simulink model "nms_model"  (R2020a)
settings: Solver=ode15s  StartTime=0.0  StopTime=2.6  MaxStep=.01  RelTol=1e-4  AbsTol=1e-6  EnableMultiTasking=on
values from neighbouring files (symbols this model uses):
  dt_visual = -1    [NMScontrol.m]    (also in runmodel.m = 0.001)
  g = params.g    [NMPCcostFunction.m]    (also in dynamicsNMPC.m = 9.81)
  m = parametersOpt(1)    [CGBgreybox.m]    (also in NMPCcostFunction.m = params.m)
undefined symbols (not defined in the file or in its folder): hatLeftHipToCenterDistWidth, initialTargetAngle, LongDelay, LongLoopDelay, LPreStimBFSHinit, LPreStimGASinit, LPreStimGLUinit, LPreStimHABinit, LPreStimHADinit, LPreStimHAMinit, LPreStimHFLinit, LPreStimRFinit, LPreStimSOLinit, LPreStimTAinit, LPreStimVASinit, LTargetAngleInit, LTargetAngleRInit, MidDelay, RPreStimBFSHinit, RPreStimGASinit, RPreStimGLUinit, RPreStimHABinit, RPreStimHADinit, RPreStimHAMinit, RPreStimHFLinit, RPreStimRFinit, RPreStimSOLinit, RPreStimTAinit, RPreStimVASinit, RTargetAngleInit, RTargetAngleRInit, ShortDelay, termination_height, thetaHATref, X, Y, Z
libraries: NeuroMuscularLibrary x107, nesl_utility x25, sm_lib x16, simulink x3
(part 2 of 3)

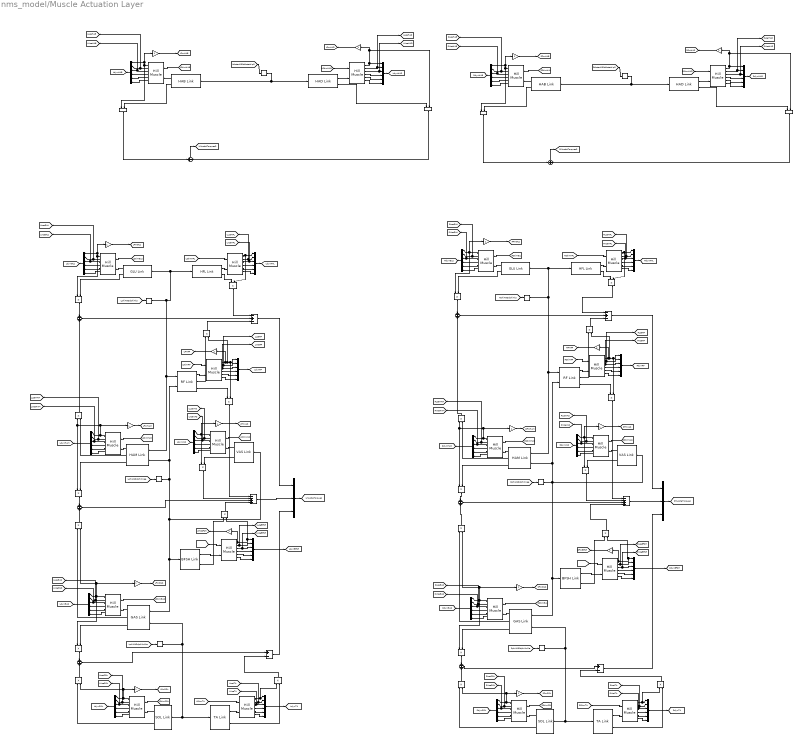
== system nms_model/Muscle Actuation Layer ==
  note: Right Hip Joint
  note: Right Knee Joint
  note: Right Ankle Joint
  note: Left Hip Joint
  note: Left Knee Joint
  note: Left Ankle Joint
  note: Left Leg
  note: Right Leg
  note: Body Mechanics Layer
      | Interface (Left Hip Joint)
  note: Muscle Actuation Layer
      | (Coronal Plane)
  note: Muscle Actuation Layer
      | (Sagittal Plane)
  note: Body Mechanics Layer
      | Interface (Right Hip Joint)
  Add1 : Sum  Inputs=-+-
  Add2 : Sum  Inputs=-+-
  Add3 : Sum  Inputs=--++
  Add4 : Sum  Inputs=+-
  Add5 : Sum  Inputs=--++
  Add6 : Sum  Inputs=+-
  L  TA Link : NeuroMuscularLibrary/TA Link  SystemSampleTime=-1  Latency=0  AutoFrameSizeCalculation=off
  L BFSH Golgi Tendon Organs : Gain
  L BFSH Link : NeuroMuscularLibrary/BFSH Link  SystemSampleTime=-1  Latency=0  AutoFrameSizeCalculation=off
  L BFSH Muscle : NeuroMuscularLibrary/Hill Muscle  Fmax=FmaxBFSH  lopt=loptBFSH  vmax=vmaxBFSH  lslack=lslackBFSH
  L GAS Golgi Tendon Organs : Gain
  L GAS Link : NeuroMuscularLibrary/GAS Link  SystemSampleTime=-1  Latency=0  AutoFrameSizeCalculation=off
  L GAS Muscle : NeuroMuscularLibrary/Hill Muscle  Fmax=FmaxGAS  lopt=loptGAS  vmax=vmaxGAS  lslack=lslackGAS
  L GLU Golgi Tendon Organs : Gain
  L GLU Link : NeuroMuscularLibrary/GLU Link  SystemSampleTime=-1  Latency=0  AutoFrameSizeCalculation=off
  L GLU Muscle : NeuroMuscularLibrary/Hill Muscle  Fmax=FmaxGLU  lopt=loptGLU  vmax=vmaxGLU  lslack=lslackGLU
  L HAB Golgi Tendon Organs : Gain
  L HAB Link : NeuroMuscularLibrary/HAB Link  SystemSampleTime=-1  Latency=0  AutoFrameSizeCalculation=off
  L HAB Muscle : NeuroMuscularLibrary/Hill Muscle  Fmax=FmaxHAB  lopt=loptHAB  vmax=vmaxHAB  lslack=lslackHAB
  L HAD Golgi Tendon Organs : Gain
  L HAD Link : NeuroMuscularLibrary/HAD Link  SystemSampleTime=-1  Latency=0  AutoFrameSizeCalculation=off
  L HAD Muscle : NeuroMuscularLibrary/Hill Muscle  Fmax=FmaxHAD  lopt=loptHAD  vmax=vmaxHAD  lslack=lslackHAD
  L HAM Golgi Tendon Organs : Gain
  L HAM Link : NeuroMuscularLibrary/HAM Link  SystemSampleTime=-1  Latency=0  AutoFrameSizeCalculation=off
  L HAM Muscle : NeuroMuscularLibrary/Hill Muscle  Fmax=FmaxHAM  lopt=loptHAM  vmax=vmaxHAM  lslack=lslackHAM
  L HFL Link : NeuroMuscularLibrary/HFL Link  SystemSampleTime=-1  Latency=0  AutoFrameSizeCalculation=off
  L HFL Muscle : NeuroMuscularLibrary/Hill Muscle  Fmax=FmaxHFL  lopt=loptHFL  vmax=vmaxHFL  lslack=lslackHFL
  L RF Golgi Tendon Organs : Gain
  L RF Link : NeuroMuscularLibrary/RF Link  SystemSampleTime=-1  Latency=0  AutoFrameSizeCalculation=off
  L RF Muscle : NeuroMuscularLibrary/Hill Muscle  Fmax=FmaxRF  lopt=loptRF  vmax=vmaxRF  lslack=lslackRF
  L SOL Golgi Tendon Organs : Gain
  L SOL Link : NeuroMuscularLibrary/SOL Link  SystemSampleTime=-1  Latency=0  AutoFrameSizeCalculation=off
  L SOL Muscle : NeuroMuscularLibrary/Hill Muscle  Fmax=FmaxSOL  lopt=loptSOL  vmax=vmaxSOL  lslack=lslackSOL
  L TA Muscle : NeuroMuscularLibrary/Hill Muscle  Fmax=FmaxTA  lopt=loptTA  vmax=vmaxTA  lslack=lslackTA
  L VAS Golgi Tendon Organs : Gain
  L VAS Link : NeuroMuscularLibrary/VAS Link  SystemSampleTime=-1  Latency=0  AutoFrameSizeCalculation=off
  L VAS Muscle : NeuroMuscularLibrary/Hill Muscle  Fmax=FmaxVAS  lopt=loptVAS  vmax=vmaxVAS  lslack=lslackVAS
  Mux : Mux  Inputs=3
  Mux1 : Mux  Inputs=3
  Mux{2..23} (22 alike) : Mux  Inputs=6
  Product{1..2,26..27} (4 alike) : Product  RndMeth=Zero
  R  TA Link : NeuroMuscularLibrary/TA Link  SystemSampleTime=-1  Latency=0  AutoFrameSizeCalculation=off
  R BFSH Golgi Tendon Organs : Gain
  R BFSH Link : NeuroMuscularLibrary/BFSH Link  SystemSampleTime=-1  Latency=0  AutoFrameSizeCalculation=off
  R BFSH Muscle : NeuroMuscularLibrary/Hill Muscle  Fmax=FmaxBFSH  lopt=loptBFSH  vmax=vmaxBFSH  lslack=lslackBFSH
  R GAS Golgi Tendon Organs : Gain
  R GAS Link : NeuroMuscularLibrary/GAS Link  SystemSampleTime=-1  Latency=0  AutoFrameSizeCalculation=off
  R GAS Muscle : NeuroMuscularLibrary/Hill Muscle  Fmax=FmaxGAS  lopt=loptGAS  vmax=vmaxGAS  lslack=lslackGAS
  R GLU Golgi Tendon Organs : Gain
  R GLU Link : NeuroMuscularLibrary/GLU Link  SystemSampleTime=-1  Latency=0  AutoFrameSizeCalculation=off
  R GLU Muscle : NeuroMuscularLibrary/Hill Muscle  Fmax=FmaxGLU  lopt=loptGLU  vmax=vmaxGLU  lslack=lslackGLU
  R HAB Golgi Tendon Organs : Gain
  R HAB Link : NeuroMuscularLibrary/HAB Link  SystemSampleTime=-1  Latency=0  AutoFrameSizeCalculation=off
  R HAB Muscle : NeuroMuscularLibrary/Hill Muscle  Fmax=FmaxHAB  lopt=loptHAB  vmax=vmaxHAB  lslack=lslackHAB
  R HAD Golgi Tendon Organs : Gain
  R HAD Link : NeuroMuscularLibrary/HAD Link  SystemSampleTime=-1  Latency=0  AutoFrameSizeCalculation=off
  R HAD Muscle : NeuroMuscularLibrary/Hill Muscle  Fmax=FmaxHAD  lopt=loptHAD  vmax=vmaxHAD  lslack=lslackHAD
  R HAM Golgi Tendon Organs : Gain
  R HAM Link : NeuroMuscularLibrary/HAM Link  SystemSampleTime=-1  Latency=0  AutoFrameSizeCalculation=off
  R HAM Muscle : NeuroMuscularLibrary/Hill Muscle  Fmax=FmaxHAM  lopt=loptHAM  vmax=vmaxHAM  lslack=lslackHAM
  R HFL Link : NeuroMuscularLibrary/HFL Link  SystemSampleTime=-1  Latency=0  AutoFrameSizeCalculation=off
  R HFL Muscle : NeuroMuscularLibrary/Hill Muscle  Fmax=FmaxHFL  lopt=loptHFL  vmax=vmaxHFL  lslack=lslackHFL
  R RF Golgi Tendon Organs : Gain
  R RF Link : NeuroMuscularLibrary/RF Link  SystemSampleTime=-1  Latency=0  AutoFrameSizeCalculation=off
  R RF Muscle : NeuroMuscularLibrary/Hill Muscle  Fmax=FmaxRF  lopt=loptRF  vmax=vmaxRF  lslack=lslackRF
  R SOL Golgi Tendon Organs : Gain
  R SOL Link : NeuroMuscularLibrary/SOL Link  SystemSampleTime=-1  Latency=0  AutoFrameSizeCalculation=off
  R SOL Muscle : NeuroMuscularLibrary/Hill Muscle  Fmax=FmaxSOL  lopt=loptSOL  vmax=vmaxSOL  lslack=lslackSOL
  R TA Muscle : NeuroMuscularLibrary/Hill Muscle  Fmax=FmaxTA  lopt=loptTA  vmax=vmaxTA  lslack=lslackTA
  R VAS Golgi Tendon Organs : Gain
  R VAS Link : NeuroMuscularLibrary/VAS Link  SystemSampleTime=-1  Latency=0  AutoFrameSizeCalculation=off
  R VAS Muscle : NeuroMuscularLibrary/Hill Muscle  Fmax=FmaxVAS  lopt=loptVAS  vmax=vmaxVAS  lslack=lslackVAS
  Selector{1..8} (8 alike) : Selector  InputPortWidth=2  IndexOptions=Index vector (dialog)  Indices=1  OutputSizes=1
  Sum{1,3..4,8,11,15} (6 alike) : Sum  Inputs=+|+
  Sum2 : Sum  Inputs=+-
  Sum25 : Sum  Inputs=+-
  tau = r*F{1..24} (24 alike) : Product
  tag scope: LFmBFSH=global, LFmGAS=global, LFmGLU=global, LFmHAB=global, LFmHAD=global, LFmHAM=global, LFmRF=global, LFmSOL=global, LFmVAS=global, LLceBFSH=global, LLceGAS=global, LLceGLU=global, LLceHAB=global, LLceHAD=global, LLceHAM=global, LLceHFL=global, LLceRF=global, LLceSOL=global, LLceTA=global, LLceVAS=global, LMuscleTorques=global, LMuscleTorquesR=global, LVceBFSH=global, LVceGAS=global, LVceGLU=global, LVceHAB=global, LVceHAD=global, LVceHAM=global, LVceHFL=global, LVceRF=global, LVceSOL=global, LVceTA=global, LVceVAS=global, LdynBFSH=global, LdynGAS=global, LdynGLU=global, LdynHAB=global, LdynHAD=global, LdynHAM=global, LdynHFL=global, LdynRF=global, LdynSOL=global, LdynTA=global, LdynVAS=global, RFmBFSH=global, RFmGAS=global, RFmGLU=global, RFmHAB=global, RFmHAD=global, RFmHAM=global, RFmRF=global, RFmSOL=global, RFmVAS=global, RLceBFSH=global, RLceGAS=global, RLceGLU=global, RLceHAB=global, RLceHAD=global, RLceHAM=global, RLceHFL=global, RLceRF=global, RLceSOL=global, RLceTA=global, RLceVAS=global, RMuscleTorques=global, RMuscleTorquesR=global, RVceBFSH=global, RVceGAS=global, RVceGLU=global, RVceHAB=global, RVceHAD=global, RVceHAM=global, RVceHFL=global, RVceRF=global, RVceSOL=global, RVceTA=global, RVceVAS=global, RdynBFSH=global, RdynGAS=global, RdynGLU=global, RdynHAB=global, RdynHAD=global, RdynHAM=global, RdynHFL=global, RdynRF=global, RdynSOL=global, RdynTA=global, RdynVAS=global
  wires:
  R HAM Link/1 -> R HAM Muscle/2
  R HAM Link/2 -> tau = r*F9/2
  R HAM Muscle/5 -> Mux7/5
  Mux7/1 -> [RdynHAM]
  R HAM Muscle/3 -> [RVceHAM], Mux7/3
  R HAM Muscle/4 -> Mux7/4
  [RphiANDdphiHip] -> Selector1/1
  Selector1/1 -> R RF Link/1, R HAM Link/1, R GLU Link/1, R HFL Link/1
  Add2/1 -> Mux/1
  R GLU Link/1 -> R GLU Muscle/2
  [RStimGLU] -> R GLU Muscle/1
  R GLU Muscle/5 -> Mux9/5
  R GLU Muscle/2 -> [RLceGLU], Mux9/2
  R GLU Muscle/3 -> [RVceGLU], Mux9/3
  R GLU Muscle/4 -> Mux9/4
  R GLU Link/2 -> tau = r*F10/2
  R GLU Muscle/1 -> Mux9/1, R GLU Golgi Tendon Organs/1, tau = r*F10/1
  R GLU Golgi Tendon Organs/1 -> [RFmGLU]
  R HFL Link/1 -> R HFL Muscle/2
  [RStimHFL] -> R HFL Muscle/1
  R HFL Muscle/5 -> Mux10/5
  Mux10/1 -> [RdynHFL]
  R HFL Muscle/4 -> Mux10/4
  R HFL Muscle/3 -> [RVceHFL], Mux10/3
  R HFL Link/2 -> tau = r*F11/1
  R HFL Muscle/1 -> Mux10/1, tau = r*F11/2
  R HAM Golgi Tendon Organs/1 -> [RFmHAM]
  [RStimHAM] -> R HAM Muscle/1
  R VAS Link/1 -> R VAS Muscle/2
  R VAS Muscle/5 -> Mux11/5
  Mux11/1 -> [RdynVAS]
  R VAS Muscle/2 -> [RLceVAS], Mux11/2
  R VAS Muscle/3 -> [RVceVAS], Mux11/3
  R VAS Muscle/4 -> Mux11/4
  R VAS Muscle/1 -> R VAS Golgi Tendon Organs/1, Mux11/1, tau = r*F13/1
  R VAS Golgi Tendon Organs/1 -> [RFmVAS]
  R VAS Link/2 -> tau = r*F13/2
  R HAM Link/3 -> tau = r*F14/2
  Sum11/1 -> Add3/3  "Knee Flexion Torque"
  [RStimVAS] -> R VAS Muscle/1
  [RphiANDdphiKnee] -> Selector3/1
  R SOL Muscle/1 -> R SOL Golgi Tendon Organs/1, tau = r*F12/2, Mux13/1
  R SOL Muscle/5 -> Mux13/5
  Mux13/1 -> [RdynSOL]
  R SOL Muscle/2 -> [RLceSOL], Mux13/2
  R SOL Muscle/3 -> [RVceSOL], Mux13/3
  R SOL Muscle/4 -> Mux13/4
  R SOL Link/2 -> tau = r*F12/1
  R SOL Link/1 -> R SOL Muscle/2
  R SOL Golgi Tendon Organs/1 -> [RFmSOL]
  [RStimSOL] -> R SOL Muscle/1
  Selector2/1 -> R GAS Link/2, R  TA Link/1, R SOL Link/1
  [RphiANDdphiAnkle] -> Selector2/1
  Add4/1 -> Mux/3
  R  TA Link/1 -> R TA Muscle/2
  R TA Muscle/1 -> tau = r*F15/1, Mux14/1
  R TA Muscle/5 -> Mux14/5
  Mux14/1 -> [RdynTA]
  R TA Muscle/4 -> Mux14/4
  R TA Muscle/3 -> Mux14/3, [RVceTA]
  [RStimTA] -> R TA Muscle/1
  R  TA Link/2 -> tau = r*F15/2
  tau = r*F15/1 -> Add4/2
  R GAS Link/1 -> R GAS Muscle/2
  Selector3/1 -> R RF Link/2, R HAM Link/2, R VAS Link/1, R GAS Link/1, R BFSH Link/1
  R GAS Muscle/5 -> Mux12/5
  Mux12/1 -> [RdynGAS]
  R GAS Muscle/2 -> [RLceGAS], Mux12/2
  R GAS Muscle/3 -> [RVceGAS], Mux12/3
  R GAS Muscle/4 -> Mux12/4
  R GAS Link/2 -> tau = r*F16/1
  [RStimGAS] -> R GAS Muscle/1
  tau = r*F12/1 -> Sum15/2
  Sum15/1 -> Add4/1
  R GAS Link/3 -> tau = r*F17/2
  tau = r*F17/1 -> Sum15/1
  R GAS Muscle/1 -> Mux12/1, tau = r*F16/2, R GAS Golgi Tendon Organs/1, tau = r*F17/1
  R GAS Golgi Tendon Organs/1 -> [RFmGAS]
  tau = r*F9/1 -> Sum8/2  "HAM"
  tau = r*F10/1 -> Sum8/1  "GLU"
  tau = r*F11/1 -> Add2/1  "HFL"
  R HAM Muscle/1 -> tau = r*F14/1, tau = r*F9/1, R HAM Golgi Tendon Organs/1, Mux7/1
  Sum8/1 -> Add2/2  "Hip Extension Moment"
  tau = r*F16/1 -> Sum11/2  "GAS"
  tau = r*F14/1 -> Sum11/1  "HAM"
  tau = r*F13/1 -> Add3/2  "VAS"
  R TA Muscle/2 -> [RLceTA], Mux14/2
  Mux9/1 -> [RdynGLU]
  Mux/1 -> [RMuscleTorques]
  L HAM Link/1 -> L HAM Muscle/2
  L HAM Link/2 -> tau = r*F18/2
  L HAM Muscle/5 -> Mux8/5
  Mux8/1 -> [LdynHAM]
  L HAM Muscle/3 -> [LVceHAM], Mux8/3
  L HAM Muscle/4 -> Mux8/4
  [LphiANDdphiHip] -> Selector4/1
  Selector4/1 -> L GLU Link/1, L HFL Link/1, L RF Link/1, L HAM Link/1
  Add1/1 -> Mux1/1
  L GLU Link/1 -> L GLU Muscle/2
  [LStimGLU] -> L GLU Muscle/1
  L GLU Muscle/5 -> Mux15/5
  L GLU Muscle/2 -> Mux15/2, [LLceGLU]
  L GLU Muscle/3 -> Mux15/3, [LVceGLU]
  L GLU Muscle/4 -> Mux15/4
  L GLU Link/2 -> tau = r*F1/2
  L GLU Muscle/1 -> Mux15/1, L GLU Golgi Tendon Organs/1, tau = r*F1/1
  L GLU Golgi Tendon Organs/1 -> [LFmGLU]
  L HFL Link/1 -> L HFL Muscle/2
  [LStimHFL] -> L HFL Muscle/1
  L HFL Muscle/5 -> Mux2/5
  Mux2/1 -> [LdynHFL]
  L HFL Muscle/4 -> Mux2/4
  L HFL Muscle/3 -> [LVceHFL], Mux2/3
  L HFL Link/2 -> tau = r*F2/1
  L HFL Muscle/1 -> Mux2/1, tau = r*F2/2
  L HAM Golgi Tendon Organs/1 -> [LFmHAM]
  [LStimHAM] -> L HAM Muscle/1
  L VAS Link/1 -> L VAS Muscle/2
  L VAS Muscle/5 -> Mux3/5
  Mux3/1 -> [LdynVAS]
  L VAS Muscle/2 -> [LLceVAS], Mux3/2
  L VAS Muscle/3 -> [LVceVAS], Mux3/3
  L VAS Muscle/4 -> Mux3/4
  L VAS Muscle/1 -> L VAS Golgi Tendon Organs/1, Mux3/1, tau = r*F4/1
  L VAS Golgi Tendon Organs/1 -> [LFmVAS]
  L VAS Link/2 -> tau = r*F4/2
  L HAM Link/3 -> tau = r*F5/2
  Sum1/1 -> Add5/3  "Knee Flexion Torque"
  [LStimVAS] -> L VAS Muscle/1
  [LphiANDdphiKnee] -> Selector6/1
  L SOL Muscle/1 -> L SOL Golgi Tendon Organs/1, tau = r*F3/2, Mux5/1
  L SOL Muscle/5 -> Mux5/5
  Mux5/1 -> [LdynSOL]
  L SOL Muscle/3 -> [LVceSOL], Mux5/3
  L SOL Muscle/4 -> Mux5/4
  L SOL Link/2 -> tau = r*F3/1
  L SOL Link/1 -> L SOL Muscle/2
  L SOL Golgi Tendon Organs/1 -> [LFmSOL]
  [LStimSOL] -> L SOL Muscle/1
  Selector5/1 -> L GAS Link/2, L  TA Link/1, L SOL Link/1
  [LphiANDdphiAnkle] -> Selector5/1
  Add6/1 -> Mux1/3
  L  TA Link/1 -> L TA Muscle/2
  L TA Muscle/1 -> tau = r*F6/1, Mux6/1
  L TA Muscle/5 -> Mux6/5
  Mux6/1 -> [LdynTA]
  L TA Muscle/4 -> Mux6/4
  L TA Muscle/3 -> Mux6/3, [LVceTA]
  [LStimTA] -> L TA Muscle/1
  L  TA Link/2 -> tau = r*F6/2
  tau = r*F6/1 -> Add6/2
  L GAS Link/1 -> L GAS Muscle/2
  Selector6/1 -> L GAS Link/1, L BFSH Link/1, L VAS Link/1, L RF Link/2, L HAM Link/2
  L GAS Muscle/5 -> Mux4/5
  Mux4/1 -> [LdynGAS]
  L GAS Muscle/2 -> [LLceGAS], Mux4/2
  L GAS Muscle/3 -> [LVceGAS], Mux4/3
  L GAS Muscle/4 -> Mux4/4
  L GAS Link/2 -> tau = r*F7/1
  [LStimGAS] -> L GAS Muscle/1
  tau = r*F3/1 -> Sum3/2
  Sum3/1 -> Add6/1
  L GAS Link/3 -> tau = r*F8/2
  tau = r*F8/1 -> Sum3/1
  L GAS Muscle/1 -> Mux4/1, tau = r*F7/2, L GAS Golgi Tendon Organs/1, tau = r*F8/1
  L GAS Golgi Tendon Organs/1 -> [LFmGAS]
  tau = r*F18/1 -> Sum4/2  "HAM"
  tau = r*F1/1 -> Sum4/1  "GLU"
  tau = r*F2/1 -> Add1/1  "HFL"
  L HAM Muscle/1 -> tau = r*F5/1, tau = r*F18/1, L HAM Golgi Tendon Organs/1, Mux8/1
  Sum4/1 -> Add1/2  "Hip Extension Moment"
  tau = r*F7/1 -> Sum1/2  "GAS"
  tau = r*F5/1 -> Sum1/1  "HAM"
  tau = r*F4/1 -> Add5/2  "VAS"
  L TA Muscle/2 -> [LLceTA], Mux6/2
  Mux15/1 -> [LdynGLU]
  Mux1/1 -> [LMuscleTorques]
  L GLU Muscle/6 -> Mux15/6
  L HFL Muscle/6 -> Mux2/6
  L HAM Muscle/6 -> Mux8/6
  L VAS Muscle/6 -> Mux3/6
  L GAS Muscle/6 -> Mux4/6
  L SOL Muscle/6 -> Mux5/6
  L TA Muscle/6 -> Mux6/6
  R SOL Muscle/6 -> Mux13/6
  R TA Muscle/6 -> Mux14/6
  R GAS Muscle/6 -> Mux12/6
  R HAM Muscle/6 -> Mux7/6
  R VAS Muscle/6 -> Mux11/6
  R HFL Muscle/6 -> Mux10/6
  R GLU Muscle/6 -> Mux9/6
  R HFL Muscle/2 -> [RLceHFL], Mux10/2
  R HAM Muscle/2 -> [RLceHAM], Mux7/2
  L HFL Muscle/2 -> [LLceHFL], Mux2/2
  L HAM Muscle/2 -> [LLceHAM], Mux8/2
  L SOL Muscle/2 -> [LLceSOL], Mux5/2
  L BFSH Muscle/3 -> [LVceBFSH], Mux16/3
  [LStimBFSH] -> L BFSH Muscle/1
  L BFSH Link/2 -> tau = r*F19/1
  L BFSH Golgi Tendon Organs/1 -> [LFmBFSH]
  L BFSH Muscle/6 -> Mux16/6
  L BFSH Muscle/4 -> Mux16/4
  L BFSH Link/1 -> L BFSH Muscle/2
  Mux16/1 -> [LdynBFSH]
  L BFSH Muscle/2 -> [LLceBFSH], Mux16/2
  L BFSH Muscle/5 -> Mux16/5
  L BFSH Muscle/1 -> tau = r*F19/2, Mux16/1, L BFSH Golgi Tendon Organs/1
  tau = r*F19/1 -> Add5/4  "BFSH"
  L RF Muscle/3 -> [LVceRF], Mux17/3
  [LStimRF] -> L RF Muscle/1
  L RF Link/3 -> tau = r*F20/2
  L RF Golgi Tendon Organs/1 -> [LFmRF]
  L RF Muscle/6 -> Mux17/6
  L RF Muscle/4 -> Mux17/4
  L RF Link/1 -> L RF Muscle/2
  Mux17/1 -> [LdynRF]
  L RF Muscle/2 -> [LLceRF], Mux17/2
  L RF Muscle/5 -> Mux17/5
  L RF Muscle/1 -> tau = r*F21/2, Mux17/1, tau = r*F20/1, L RF Golgi Tendon Organs/1
  L RF Link/2 -> tau = r*F21/1
  tau = r*F21/1 -> Add1/3  "RF"
  tau = r*F20/1 -> Add5/1  "RF"
  R BFSH Muscle/3 -> [RVceBFSH], Mux18/3
  [RStimBFSH] -> R BFSH Muscle/1
  R BFSH Muscle/1 -> tau = r*F22/2, Mux18/1, R BFSH Golgi Tendon Organs/1
  R BFSH Muscle/4 -> Mux18/4
  R BFSH Golgi Tendon Organs/1 -> [RFmBFSH]
  R BFSH Muscle/5 -> Mux18/5
  Mux18/1 -> [RdynBFSH]
  R BFSH Muscle/2 -> [RLceBFSH], Mux18/2
  R BFSH Link/1 -> R BFSH Muscle/2
  R BFSH Link/2 -> tau = r*F22/1
  R BFSH Muscle/6 -> Mux18/6
  tau = r*F22/1 -> Add3/4  "BFSH"
  [RStimRF] -> R RF Muscle/1
  R RF Muscle/3 -> [RVceRF], Mux19/3
  R RF Muscle/4 -> Mux19/4
  R RF Muscle/6 -> Mux19/6
  R RF Muscle/5 -> Mux19/5
  R RF Muscle/2 -> [RLceRF], Mux19/2
  R RF Muscle/1 -> tau = r*F24/2, Mux19/1, tau = r*F23/1, R RF Golgi Tendon Organs/1
  Mux19/1 -> [RdynRF]
  R RF Link/3 -> tau = r*F23/2
  R RF Link/2 -> tau = r*F24/1
  R RF Golgi Tendon Organs/1 -> [RFmRF]
  R RF Link/1 -> R RF Muscle/2
  tau = r*F24/1 -> Add2/3  "RF"
  tau = r*F23/1 -> Add3/1  "RF"
  Product27/1 -> Sum25/2
  L HAD Link/2 -> Product27/1
  Selector7/1 -> L HAB Link/1, L HAD Link/1
  Product26/1 -> Sum25/1
  L HAB Muscle/6 -> Mux20/6
  L HAB Muscle/1 -> Product26/1, Mux20/1, L HAB Golgi Tendon Organs/1
  L HAB Golgi Tendon Organs/1 -> [LFmHAB]
  L HAB Muscle/4 -> Mux20/4
  L HAB Muscle/2 -> Mux20/2, [LLceHAB]
  L HAB Muscle/5 -> Mux20/5
  L HAB Link/1 -> L HAB Muscle/2
  L HAB Link/2 -> Product26/2
  L HAB Muscle/3 -> Mux20/3, [LVceHAB]
  [LStimHAB] -> L HAB Muscle/1
  Mux20/1 -> [LdynHAB]
  [LthetaANDdthetaHipR] -> Selector7/1
  L HAD Link/1 -> L HAD Muscle/2
  [LStimHAD] -> L HAD Muscle/1
  L HAD Golgi Tendon Organs/1 -> [LFmHAD]
  L HAD Muscle/2 -> Mux21/2, [LLceHAD]
  L HAD Muscle/1 -> Mux21/1, Product27/2, L HAD Golgi Tendon Organs/1
  L HAD Muscle/3 -> [LVceHAD], Mux21/3
  L HAD Muscle/4 -> Mux21/4
  L HAD Muscle/5 -> Mux21/5
  L HAD Muscle/6 -> Mux21/6
  Mux21/1 -> [LdynHAD]
  Sum25/1 -> [LMuscleTorquesR]
  R HAD Muscle/6 -> Mux23/6
  Selector8/1 -> R HAB Link/1, R HAD Link/1
  R HAD Link/2 -> Product2/1
  R HAD Golgi Tendon Organs/1 -> [RFmHAD]
  [RStimHAD] -> R HAD Muscle/1
  Mux23/1 -> [RdynHAD]
  Sum2/1 -> [RMuscleTorquesR]
  Mux22/1 -> [RdynHAB]
  R HAB Golgi Tendon Organs/1 -> [RFmHAB]
  Product1/1 -> Sum2/1
  Product2/1 -> Sum2/2
  R HAD Muscle/5 -> Mux23/5
  R HAD Muscle/2 -> Mux23/2, [RLceHAD]
  R HAD Muscle/3 -> [RVceHAD], Mux23/3
  R HAD Link/1 -> R HAD Muscle/2
  [RthetaANDdthetaHipR] -> Selector8/1
  R HAD Muscle/1 -> Mux23/1, Product2/2, R HAD Golgi Tendon Organs/1
  R HAB Link/2 -> Product1/2
  R HAB Muscle/5 -> Mux22/5
  R HAB Muscle/2 -> Mux22/2, [RLceHAB]
  R HAD Muscle/4 -> Mux23/4
  R HAB Link/1 -> R HAB Muscle/2
  R HAB Muscle/4 -> Mux22/4
  R HAB Muscle/3 -> Mux22/3, [RVceHAB]
  R HAB Muscle/6 -> Mux22/6
  R HAB Muscle/1 -> Product1/1, Mux22/1, R HAB Golgi Tendon Organs/1
  [RStimHAB] -> R HAB Muscle/1
  Add5/1 -> Mux1/2
  Add3/1 -> Mux/2

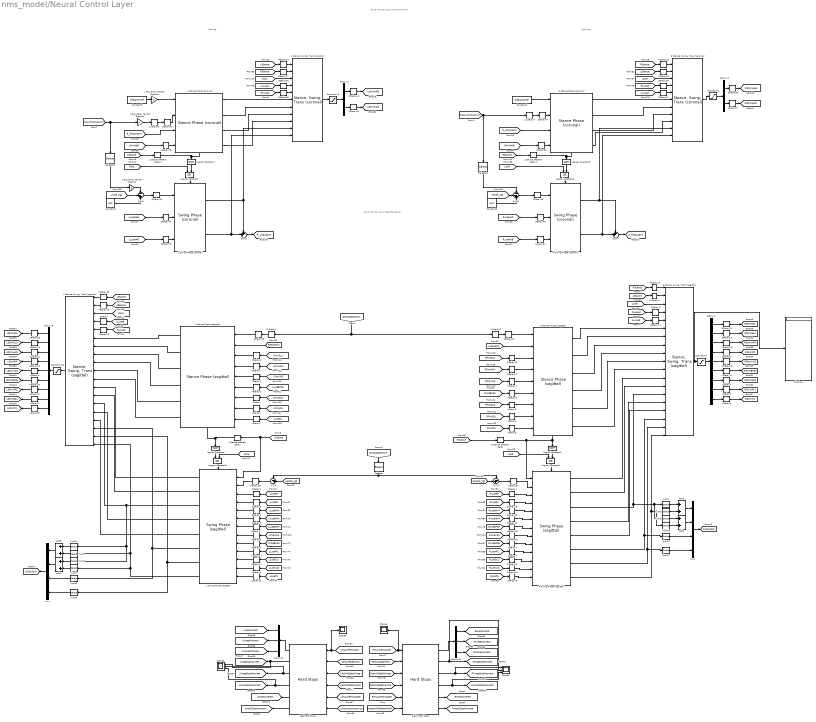
== system nms_model/Neural Control Layer ==
  note: Neural Control Layer
      | (Sagittal Plane)
  note: Neural Control Layer
      | (Coronal Plane)
  note: Right Leg
  note: Left Leg
  Add{1..3,9} (4 alike) : Sum  Inputs=2
  Constant1 : Constant  Value=pi/2
  Constant2 : Constant  Value=pi/2
  Constant3 : Constant  Value=thetaHATref
  Constant4 : Constant  Value=thetaHATref
  Demux1 : Demux  Outputs=2
  Demux10 : Demux  Outputs=3
  Demux2 : Demux  Outputs=2
  Demux6 : Demux  Outputs=9
  Demux7 : Demux  Outputs=9
  Demux8 : Demux  Outputs=3
  Display1 : Display
  L GLU Golgi Tendon Organs1 : Gain  Gain=-1
  L GLU Golgi Tendon Organs2 : Gain  Gain=-1
  L GLU Golgi Tendon Organs3 : Gain  Gain=-1
  L Stance afferent delay : TransportDelay  DelayTime=MidDelay
  L Stance afferent delay1 : TransportDelay  DelayTime=MidDelay
  L Stance afferent delay2 : TransportDelay  DelayTime=MidDelay
  L Stance Phase (coronal) : NeuroMuscularLibrary/Stance Phase (coronal)  PreStimHABst=PreStimHABst  PreStimHADst=PreStimHADst  GainFHABst=GainFHABst  GainPhiHATHABst=GainPhiHATHABst  GainDphiHATHABst=GainDphiHATHABst  GainPhiHATHADst=GainPhiHATHADst  GainDphiHATHADst=GainDphiHATHADst  GainSHABcHABst=GainSHABcHABst  GainSHADcHADst=GainSHADcHADst
  L Stance Phase (sagittal) : NeuroMuscularLibrary/Stance Phase (sagittal)  PreStimHFLst=PreStimHFLst  PreStimGLUst=PreStimGLUst  PreStimHAMst=PreStimHAMst  PreStimRFst=PreStimRFst  PreStimVASst=PreStimVASst  PreStimBFSHst=PreStimBFSHst  PreStimGASst=PreStimGASst  PreStimSOLst=PreStimSOLst  PreStimTAst=PreStimTAst  GainFGLUst=GainFGLUst  GainFVASst=GainFVASst  GainFSOLst=GainFSOLst  GainFHAMst=GainFHAMst  LceOffsetBFSHVASst=LceOffsetBFSHVASst  GainLBFSHVASst=GainLBFSHVASst  LceOffsetBFSHst=LceOffsetBFSHst  GainLBFSHst=GainLBFSHst  GainFGASst=GainFGASst  phiHATref=phiHATref  GainPhiHATHFLst=GainPhiHATHFLst  GainDphiHATHFLst=GainDphiHATHFLst  GainPhiHATGLUst=GainPhiHATGLUst  GainDphiHATGLUst=GainDphiHATGLUst  GainSGLUHAMst=GainSGLUHAMst  GainSGLUcHFLst=GainSGLUcHFLst  GainSHAMcHFLst=GainSHAMcHFLst  GainSHFLcGLUst=GainSHFLcGLUst  GainSRFcGLUst=GainSRFcGLUst  LceOffsetTAst=LceOffsetTAst  GainLTAst=GainLTAst  GainFSOLTAst=GainFSOLTAst
  "L Stance, Swing, Trans (coronal)" : NeuroMuscularLibrary/Stance, Swing, Trans (coronal)  transSupst_C=transSupst_C  transsw_C=transsw_C
  "L Stance, Swing, Trans (sagittal)" : NeuroMuscularLibrary/Stance, Swing, Trans (sagittal)  transSupst=transSupst  transsw=transsw
  L Swing Phase (coronal) : NeuroMuscularLibrary/Swing Phase (coronal)  PreStimHABsw=PreStimHABsw  PreStimHADsw=PreStimHADsw  GainLHABsw=GainLHABsw  GainLHADsw=GainLHADsw
  L Swing Phase (sagittal) : NeuroMuscularLibrary/Swing Phase (sagittal)  PreStimHFLsw=PreStimHFLsw  PreStimGLUsw=PreStimGLUsw  PreStimHAMsw=PreStimHAMsw  PreStimRFsw=PreStimRFsw  PreStimVASsw=PreStimVASsw  PreStimBFSHsw=PreStimBFSHsw  PreStimGASsw=PreStimGASsw  PreStimSOLsw=PreStimSOLsw  PreStimTAsw=PreStimTAsw  GainLTAsw=GainLTAsw  LceOffsetTAsw=LceOffsetTAsw  GainLRFHFLsw=GainLRFHFLsw  GainVRFHFLsw=GainVRFHFLsw  GainLHAMGLUsw=GainLHAMGLUsw  GainVHAMGLUsw=GainVHAMGLUsw  GainVRFBFSHsw=GainVRFBFSHsw  GainVVASRFsw=GainVVASRFsw  GainVBFSHsw=GainVBFSHsw  GainLHAMsw=GainLHAMsw  GainSHAMBFSHsw=GainSHAMBFSHsw  GainSHAMGASsw=GainSHAMGASsw  SHAMthresholdsw=SHAMthresholdsw  GainLHFLsw=GainLHFLsw  GainLGLUsw=GainLGLUsw  LceOffsetVASsw=LceOffsetVASsw  GainLVASsw=GainLVASsw  legLengthClr=legLengthClr  deltaLegAngleThr=deltaLegAngleThr
  LDelay{,1,3..4} (4 alike) : TransportDelay  DelayTime=LongDelay
  LDelay10 : TransportDelay  DelayTime=LongDelay  InitialOutput=LPreStimTAinit
  LDelay11 : TransportDelay  DelayTime=LongDelay  InitialOutput=LPreStimGASinit
  LDelay{2,5,12..13} (4 alike) : TransportDelay  DelayTime=LongDelay  InitialOutput=1
  LDelay6 : TransportDelay  DelayTime=LongDelay  InitialOutput=RPreStimTAinit
  LDelay7 : TransportDelay  DelayTime=LongDelay  InitialOutput=RPreStimGASinit
  LDelay8 : TransportDelay  DelayTime=LongDelay  InitialOutput=RPreStimSOLinit
  LDelay9 : TransportDelay  DelayTime=LongDelay  InitialOutput=LPreStimSOLinit
  LL Delay{2..3,6..7} (4 alike) : TransportDelay  DelayTime=LongLoopDelay/2
  Left Hard Stops : NeuroMuscularLibrary/Hard Stops  SystemSampleTime=-1  Latency=0  AutoFrameSizeCalculation=off
  Logical Operator{,1,4..5} (4 alike) : Logic  Operator=NOT  AllPortsSameDT=off  OutDataTypeStr=boolean
  Logical Operator{2..3,6..7} (4 alike) : Logic  Operator=OR  AllPortsSameDT=off  OutDataTypeStr=boolean
  MDelay{1..2,4,7..8,13..14,16,19..24} (14 alike) : TransportDelay  DelayTime=MidDelay
  MDelay10 : TransportDelay  DelayTime=MidDelay  InitialOutput=LPreStimBFSHinit
  MDelay11 : TransportDelay  DelayTime=MidDelay  InitialOutput=RPreStimBFSHinit
  MDelay12 : TransportDelay  DelayTime=MidDelay  InitialOutput=RPreStimVASinit
  MDelay{3,5..6,15,17..18} (6 alike) : TransportDelay  DelayTime=MidDelay  InitialOutput=1
  MDelay9 : TransportDelay  DelayTime=MidDelay  InitialOutput=LPreStimVASinit
  Mux : Mux
  Mux1 : Mux
  R Stance afferent delay : TransportDelay  DelayTime=MidDelay
  R Stance Phase (coronal) : NeuroMuscularLibrary/Stance Phase (coronal)  PreStimHABst=PreStimHABst  PreStimHADst=PreStimHADst  GainFHABst=GainFHABst  GainPhiHATHABst=GainPhiHATHABst  GainDphiHATHABst=GainDphiHATHABst  GainPhiHATHADst=GainPhiHATHADst  GainDphiHATHADst=GainDphiHATHADst  GainSHABcHABst=GainSHABcHABst  GainSHADcHADst=GainSHADcHADst
  R Stance Phase (sagittal) : NeuroMuscularLibrary/Stance Phase (sagittal)  PreStimHFLst=PreStimHFLst  PreStimGLUst=PreStimGLUst  PreStimHAMst=PreStimHAMst  PreStimRFst=PreStimRFst  PreStimVASst=PreStimVASst  PreStimBFSHst=PreStimBFSHst  PreStimGASst=PreStimGASst  PreStimSOLst=PreStimSOLst  PreStimTAst=PreStimTAst  GainFGLUst=GainFGLUst  GainFVASst=GainFVASst  GainFSOLst=GainFSOLst  GainFHAMst=GainFHAMst  LceOffsetBFSHVASst=LceOffsetBFSHVASst  GainLBFSHVASst=GainLBFSHVASst  LceOffsetBFSHst=LceOffsetBFSHst  GainLBFSHst=GainLBFSHst  GainFGASst=GainFGASst  phiHATref=phiHATref  GainPhiHATHFLst=GainPhiHATHFLst  GainDphiHATHFLst=GainDphiHATHFLst  GainPhiHATGLUst=GainPhiHATGLUst  GainDphiHATGLUst=GainDphiHATGLUst  GainSGLUHAMst=GainSGLUHAMst  GainSGLUcHFLst=GainSGLUcHFLst  GainSHAMcHFLst=GainSHAMcHFLst  GainSHFLcGLUst=GainSHFLcGLUst  GainSRFcGLUst=GainSRFcGLUst  LceOffsetTAst=LceOffsetTAst  GainLTAst=GainLTAst  GainFSOLTAst=GainFSOLTAst
  "R Stance, Swing, Trans (coronal)" : NeuroMuscularLibrary/Stance, Swing, Trans (coronal)  transSupst_C=transSupst_C  transsw_C=transsw_C
  "R Stance, Swing, Trans (sagittal)" : NeuroMuscularLibrary/Stance, Swing, Trans (sagittal)  transSupst=transSupst  transsw=transsw
  R Swing Phase (coronal) : NeuroMuscularLibrary/Swing Phase (coronal)  PreStimHABsw=PreStimHABsw  PreStimHADsw=PreStimHADsw  GainLHABsw=GainLHABsw  GainLHADsw=GainLHADsw
  R Swing Phase (sagittal) : NeuroMuscularLibrary/Swing Phase (sagittal)  PreStimHFLsw=PreStimHFLsw  PreStimGLUsw=PreStimGLUsw  PreStimHAMsw=PreStimHAMsw  PreStimRFsw=PreStimRFsw  PreStimVASsw=PreStimVASsw  PreStimBFSHsw=PreStimBFSHsw  PreStimGASsw=PreStimGASsw  PreStimSOLsw=PreStimSOLsw  PreStimTAsw=PreStimTAsw  GainLTAsw=GainLTAsw  LceOffsetTAsw=LceOffsetTAsw  GainLRFHFLsw=GainLRFHFLsw  GainVRFHFLsw=GainVRFHFLsw  GainLHAMGLUsw=GainLHAMGLUsw  GainVHAMGLUsw=GainVHAMGLUsw  GainVRFBFSHsw=GainVRFBFSHsw  GainVVASRFsw=GainVVASRFsw  GainVBFSHsw=GainVBFSHsw  GainLHAMsw=GainLHAMsw  GainSHAMBFSHsw=GainSHAMBFSHsw  GainSHAMGASsw=GainSHAMGASsw  SHAMthresholdsw=SHAMthresholdsw  GainLHFLsw=GainLHFLsw  GainLGLUsw=GainLGLUsw  LceOffsetVASsw=LceOffsetVASsw  GainLVASsw=GainLVASsw  legLengthClr=legLengthClr  deltaLegAngleThr=deltaLegAngleThr
  Right Hard Stops : NeuroMuscularLibrary/Hard Stops  SystemSampleTime=-1  Latency=0  AutoFrameSizeCalculation=off
  SDelay{,3,6..9,12,14,16..19,29..30,32..33,36,38..39,41..42,47} (22 alike) : TransportDelay  DelayTime=ShortDelay
  SDelay{1..2,4..5,10..11,13,15,34,44..45,49} (12 alike) : TransportDelay  DelayTime=ShortDelay  InitialOutput=1
  SDelay20 : TransportDelay  DelayTime=ShortDelay  InitialOutput=LPreStimHFLinit
  SDelay21 : TransportDelay  DelayTime=ShortDelay  InitialOutput=LPreStimGLUinit
  SDelay22 : TransportDelay  DelayTime=ShortDelay  InitialOutput=LPreStimHAMinit
  SDelay23 : TransportDelay  DelayTime=ShortDelay  InitialOutput=LPreStimRFinit
  SDelay24 : TransportDelay  DelayTime=ShortDelay  InitialOutput=RPreStimHFLinit
  SDelay25 : TransportDelay  DelayTime=ShortDelay  InitialOutput=RPreStimGLUinit
  SDelay26 : TransportDelay  DelayTime=ShortDelay  InitialOutput=RPreStimHAMinit
  SDelay27 : TransportDelay  DelayTime=ShortDelay  InitialOutput=RPreStimRFinit
  SDelay35 : TransportDelay  DelayTime=ShortDelay  InitialOutput=RPreStimHABinit
  SDelay37 : TransportDelay  DelayTime=ShortDelay  InitialOutput=RPreStimHADinit
  SDelay40 : TransportDelay  DelayTime=ShortDelay  InitialOutput=LPreStimHADinit
  SDelay43 : TransportDelay  DelayTime=(ShortDelay + LongLoopDelay/2)  InitialOutput=LTargetAngleRInit
  SDelay46 : TransportDelay  DelayTime=ShortDelay  InitialOutput=LPreStimHABinit
  SDelay48 : TransportDelay  DelayTime=(ShortDelay + LongLoopDelay/2)  InitialOutput=RTargetAngleRInit
  Saturation{1..3,10} (4 alike) : Saturate  UpperLimit=1  LowerLimit=0.01  ZeroCross=off
  Scope1 : Scope  NumInputPorts=3
  Scope2 : Scope  NumInputPorts=3
  Scope3 : Scope
  Scope4 : Scope
  Selector : Selector  InputPortWidth=2  IndexOptions=Index vector (dialog)  Indices=[1]  OutputSizes=1
  Selector1 : Selector  InputPortWidth=2  IndexOptions=Index vector (dialog)  Indices=[1]  OutputSizes=1
  Selector2 : Selector  InputPortWidth=2  IndexOptions=Index vector (dialog)  Indices=[1]  OutputSizes=1
  Sum1 : Sum  Inputs=-+|
  Sum2 : Sum  Inputs=++|
  Sum3 : Sum  Inputs=--+
  Sum4 : Sum  Inputs=++|
  Sum5 : Sum  Inputs=--+
  Sum6 : Sum  Inputs=-+|
  TDelay28 : TransportDelay  DelayTime=(ShortDelay + LongLoopDelay/2)  InitialOutput=LTargetAngleInit
  TDelay31 : TransportDelay  DelayTime=(ShortDelay + LongLoopDelay/2)  InitialOutput=RTargetAngleInit
  hipM{1,4,9,12} (4 alike) : Selector  InputPortWidth=2  IndexOptions=Index vector (dialog)  Indices=1  OutputSizes=1
  hipM10 : Selector  InputPortWidth=3  IndexOptions=Index vector (dialog)  Indices=2  OutputSizes=1
  hipM{2,5,8,11} (4 alike) : Selector  InputPortWidth=3  IndexOptions=Index vector (dialog)  Indices=1  OutputSizes=1
  hipM3 : Selector  InputPortWidth=2  IndexOptions=Index vector (dialog)  Indices=2  OutputSizes=1
  hipM6 : Selector  InputPortWidth=2  IndexOptions=Index vector (dialog)  Indices=2  OutputSizes=1
  hipM7 : Selector  InputPortWidth=3  IndexOptions=Index vector (dialog)  Indices=2  OutputSizes=1
  tag scope: LAnkleMoment=global, LAnkleStopMoment=global, LHSwStim=global, LHipMoment=global, LHipMomentR=global, LHipRStopMoment=global, LHipStopMoment=global, LKneeMoment=global, LKneeStopMoment=global, LStimBFSH=global, LStimGAS=global, LStimGLU=global, LStimHAB=global, LStimHAD=global, LStimHAM=global, LStimHFL=global, LStimRF=global, LStimSOL=global, LStimTA=global, LStimVAS=global, RAnkleMoment=global, RAnkleStopMoment=global, RHSwStim=global, RHipMoment=global, RHipMomentR=global, RHipRStopMoment=global, RHipStopMoment=global, RKneeMoment=global, RKneeStopMoment=global, RStimBFSH=global, RStimGAS=global, RStimGLU=global, RStimHAB=global, RStimHAD=global, RStimHAM=global, RStimHFL=global, RStimRF=global, RStimSOL=global, RStimTA=global, RStimVAS=global, R_LHSwStim=global, R_RHSwStim=global
  wires:
  LDelay11/1 -> [LStimGAS]
  [RLceVAS] -> MDelay15/1
  LDelay10/1 -> [LStimTA]
  L Swing Phase (sagittal)/7 -> "L Stance, Swing, Trans (sagittal)"/18, hipM8/1
  Mux/1 -> [LHSwStim]
  hipM2/1 -> Add3/2
  SDelay11/1 -> L Swing Phase (sagittal)/11
  MDelay16/1 -> R Swing Phase (sagittal)/8
  SDelay24/1 -> [RStimHFL]
  [RLceRF] -> SDelay4/1
  MDelay19/1 -> "L Stance, Swing, Trans (sagittal)"/2
  SDelay10/1 -> L Swing Phase (sagittal)/10
  hipM10/1 -> Add2/2
  R Stance Phase (sagittal)/5 -> "R Stance, Swing, Trans (sagittal)"/10
  hipM4/1 -> Add9/1
  SDelay2/1 -> L Swing Phase (sagittal)/5
  [RLceBFSH] -> MDelay6/1
  [RLceGLU] -> SDelay13/1
  L Swing Phase (sagittal)/1 -> "L Stance, Swing, Trans (sagittal)"/12
  LDelay/1 -> L Stance Phase (sagittal)/7
  L Stance Phase (sagittal)/1 -> "L Stance, Swing, Trans (sagittal)"/6
  SDelay9/1 -> L Swing Phase (sagittal)/6
  L Swing Phase (sagittal)/3 -> "L Stance, Swing, Trans (sagittal)"/14, hipM6/1, hipM4/1
  R Swing Phase (sagittal)/7 -> "R Stance, Swing, Trans (sagittal)"/18, hipM11/1
  R Swing Phase (sagittal)/4 -> "R Stance, Swing, Trans (sagittal)"/15
  Add2/1 -> Mux1/2
  L Swing Phase (sagittal)/5 -> "L Stance, Swing, Trans (sagittal)"/16
  SDelay14/1 -> "R Stance, Swing, Trans (sagittal)"/5
  Demux6/2 -> SDelay21/1
  R Stance Phase (sagittal)/2 -> "R Stance, Swing, Trans (sagittal)"/7
  SDelay12/1 -> "L Stance, Swing, Trans (sagittal)"/5
  MDelay2/1 -> L Stance Phase (sagittal)/5
  Sum1/1 -> TDelay31/1
  Demux7/8 -> LDelay8/1
  hipM6/1 -> Add1/1
  R Stance Phase (sagittal)/3 -> "R Stance, Swing, Trans (sagittal)"/8
  LDelay9/1 -> [LStimSOL]
  Demux6/1 -> SDelay20/1
  L Stance Phase (sagittal)/6 -> "L Stance, Swing, Trans (sagittal)"/11
  SDelay4/1 -> R Swing Phase (sagittal)/3
  [RVceVAS] -> MDelay16/1
  hipM11/1 -> Mux1/4
  MDelay8/1 -> L Swing Phase (sagittal)/8
  Add3/1 -> Mux1/1
  R Swing Phase (sagittal)/6 -> "R Stance, Swing, Trans (sagittal)"/17, hipM12/1
  "R Stance, Swing, Trans (sagittal)"/1 -> Display1/1, Saturation1/1
  [RVceBFSH] -> MDelay7/1
  Add1/1 -> Mux/2
  hipM9/1 -> Mux/3
  L Stance Phase (sagittal)/3 -> "L Stance, Swing, Trans (sagittal)"/8
  LDelay8/1 -> [RStimSOL]
  Logical Operator2/1 -> R Swing Phase (sagittal)/Enable
  hipM5/1 -> Add9/2
  MDelay20/1 -> "L Stance, Swing, Trans (sagittal)"/1
  L Swing Phase (sagittal)/2 -> "L Stance, Swing, Trans (sagittal)"/13
  hipM8/1 -> Mux/4
  L Swing Phase (sagittal)/4 -> "L Stance, Swing, Trans (sagittal)"/15
  L Swing Phase (sagittal)/8 -> "L Stance, Swing, Trans (sagittal)"/19, hipM5/1, hipM7/1
  [LStance] -> MDelay20/1
  R Stance Phase (sagittal)/4 -> "R Stance, Swing, Trans (sagittal)"/9
  LL Delay3/1 -> SDelay30/1
  SDelay30/1 -> R Stance Phase (sagittal)/1
  SDelay22/1 -> [LStimHAM]
  SDelay29/1 -> L Stance Phase (sagittal)/1
  TDelay28/1 -> L Swing Phase (sagittal)/2
  hipM1/1 -> Add3/1
  R Stance Phase (sagittal)/6 -> "R Stance, Swing, Trans (sagittal)"/11
  R Swing Phase (sagittal)/8 -> "R Stance, Swing, Trans (sagittal)"/19, hipM2/1, hipM10/1
  Sum6/1 -> TDelay28/1
  Demux7/1 -> SDelay24/1
  [LLceGLU] -> SDelay11/1
  [RLceHFL] -> SDelay5/1
  L Stance Phase (sagittal)/2 -> "L Stance, Swing, Trans (sagittal)"/7
  R Stance Phase (sagittal)/1 -> "R Stance, Swing, Trans (sagittal)"/6
  [LLceVAS] -> MDelay5/1
  [LHSwStim] -> R Stance Phase (sagittal)/2
  SDelay/1 -> "L Stance, Swing, Trans (sagittal)"/4
  SDelay27/1 -> [RStimRF]
  MDelay11/1 -> [RStimBFSH]
  [RFmSOL] -> LDelay4/1
  MDelay10/1 -> [LStimBFSH]
  Add9/1 -> Mux/1
  [LLceHFL] -> SDelay10/1
  SDelay26/1 -> [RStimHAM]
  SDelay21/1 -> [LStimGLU]
  Demux7/6 -> MDelay11/1
  Demux7/5 -> MDelay12/1
  [LLLoad] -> SDelay14/1
  Saturation1/1 -> Demux7/1
  SDelay5/1 -> R Swing Phase (sagittal)/10
  [LFmSOL] -> LDelay1/1
  hipM12/1 -> Mux1/3
  [LonR] -> "R Stance, Swing, Trans (sagittal)"/3
  MDelay15/1 -> R Swing Phase (sagittal)/12
  [LLLoad] -> SDelay/1
  SDelay25/1 -> [RStimGLU]
  Demux7/3 -> SDelay26/1
  L Stance Phase (sagittal)/4 -> "L Stance, Swing, Trans (sagittal)"/9
  Demux7/4 -> SDelay27/1
  hipM3/1 -> Add2/1
  R Swing Phase (sagittal)/2 -> "R Stance, Swing, Trans (sagittal)"/13
  R Swing Phase (sagittal)/1 -> "R Stance, Swing, Trans (sagittal)"/12
  L Stance Phase (sagittal)/5 -> "L Stance, Swing, Trans (sagittal)"/10
  MDelay9/1 -> [LStimVAS]
  MDelay7/1 -> R Swing Phase (sagittal)/9
  SDelay3/1 -> "R Stance, Swing, Trans (sagittal)"/4
  Demux7/9 -> LDelay6/1
  TDelay31/1 -> R Swing Phase (sagittal)/2
  SDelay19/1 -> R Swing Phase (sagittal)/6
  [RVceHAM] -> SDelay19/1
  SDelay18/1 -> R Swing Phase (sagittal)/4
  SDelay15/1 -> R Swing Phase (sagittal)/5
  [RLceHAM] -> SDelay15/1
  [RLceTA] -> LDelay5/1
  LDelay7/1 -> [RStimGAS]
  LDelay3/1 -> R Stance Phase (sagittal)/7
  [RFmGAS] -> LDelay3/1
  [LLceBFSH] -> MDelay3/1
  [RFmVAS] -> MDelay1/1
  [RLLoad] -> SDelay3/1
  SDelay17/1 -> R Stance Phase (sagittal)/4
  Demux6/7 -> LDelay11/1
  [RStance] -> MDelay19/1
  Saturation10/1 -> Demux6/1
  MDelay4/1 -> L Swing Phase (sagittal)/9
  L Swing Phase (sagittal)/6 -> "L Stance, Swing, Trans (sagittal)"/17, hipM9/1
  Demux6/6 -> MDelay10/1
  Demux6/3 -> SDelay22/1
  LDelay6/1 -> [RStimTA]
  [LVceBFSH] -> MDelay4/1
  SDelay8/1 -> L Swing Phase (sagittal)/4
  Demux6/9 -> LDelay10/1
  [RVceRF] -> SDelay18/1
  Demux6/8 -> LDelay9/1
  Demux6/5 -> MDelay9/1
  MDelay5/1 -> L Swing Phase (sagittal)/12
  SDelay16/1 -> R Stance Phase (sagittal)/3
  SDelay23/1 -> [LStimRF]
  [RLLoad] -> SDelay12/1
  R Swing Phase (sagittal)/3 -> "R Stance, Swing, Trans (sagittal)"/14, hipM3/1, hipM1/1
  [LVceRF] -> SDelay8/1
  SDelay13/1 -> R Swing Phase (sagittal)/11
  Mux1/1 -> [RHSwStim]
  LDelay4/1 -> R Stance Phase (sagittal)/8
  MDelay1/1 -> R Stance Phase (sagittal)/5
  L Stance afferent delay/1 -> L Stance Phase (sagittal)/Enable, Logical Operator/1
  Logical Operator3/1 -> L Swing Phase (sagittal)/Enable
  SDelay20/1 -> [LStimHFL]
  [LLceRF] -> SDelay1/1
  [LVceHAM] -> SDelay9/1
  LDelay2/1 -> L Stance Phase (sagittal)/9
  [LLceTA] -> LDelay2/1
  Demux7/2 -> SDelay25/1
  SDelay1/1 -> L Swing Phase (sagittal)/3
  [RFmHAM] -> SDelay17/1
  Logical Operator/1 -> Logical Operator3/2
  [LLceHAM] -> SDelay2/1
  Demux6/4 -> SDelay23/1
  LDelay1/1 -> L Stance Phase (sagittal)/8
  [LFmGAS] -> LDelay/1
  [RFmGLU] -> SDelay16/1
  MDelay3/1 -> L Stance Phase (sagittal)/6
  SDelay6/1 -> L Stance Phase (sagittal)/3
  [LVceVAS] -> MDelay8/1
  [LFmVAS] -> MDelay2/1
  LL Delay2/1 -> SDelay29/1
  Demux7/7 -> LDelay7/1
  R Swing Phase (sagittal)/5 -> "R Stance, Swing, Trans (sagittal)"/16
  [LFmGLU] -> SDelay6/1
  SDelay7/1 -> L Stance Phase (sagittal)/4
  MDelay6/1 -> R Stance Phase (sagittal)/6
  MDelay12/1 -> [RStimVAS]
  [LFmHAM] -> SDelay7/1
  [RHSwStim] -> L Stance Phase (sagittal)/2
  hipM7/1 -> Add1/2
  Logical Operator1/1 -> Logical Operator2/2
  [RLceTA] -> LDelay12/1
  LDelay12/1 -> R Swing Phase (sagittal)/13
  [LLceTA] -> LDelay13/1
  MDelay17/1 -> L Swing Phase (sagittal)/7
  [LLceBFSH] -> MDelay17/1
  LDelay13/1 -> L Swing Phase (sagittal)/13
  MDelay18/1 -> R Swing Phase (sagittal)/7
  [RLceBFSH] -> MDelay18/1
  LDelay5/1 -> R Stance Phase (sagittal)/9
  R Stance afferent delay/1 -> R Swing Phase (sagittal)/1, R Stance Phase (sagittal)/Enable, Logical Operator1/1
  [RonL] -> "L Stance, Swing, Trans (sagittal)"/3
  [LonR] -> Logical Operator2/1
  [RonL] -> Logical Operator3/1
  [RStance] -> MDelay13/1
  MDelay13/1 -> "R Stance, Swing, Trans (sagittal)"/1
  [LStance] -> MDelay14/1
  MDelay14/1 -> "R Stance, Swing, Trans (sagittal)"/2
  [Ralpha_tgt] -> Sum1/2
  Selector/1 -> Sum6/1, Sum1/1
  [Lalpha_tgt] -> Sum6/2
  [phiANDdphiHAT] -> LL Delay2/1, LL Delay3/1
  [RFmHAB] -> SDelay38/1
  SDelay35/1 -> [RStimHAB]
  [LFmHAB] -> SDelay39/1
  SDelay37/1 -> [RStimHAD]
  [LLceHAD] -> SDelay44/1
  SDelay39/1 -> L Stance Phase (coronal)/4
  L Stance Phase (coronal)/2 -> "L Stance, Swing, Trans (coronal)"/7
  MDelay21/1 -> "L Stance, Swing, Trans (coronal)"/2
  L Swing Phase (coronal)/2 -> "L Stance, Swing, Trans (coronal)"/11, Sum2/2
  [LhipR_tgt] -> Sum3/2
  L GLU Golgi Tendon Organs2/1 -> Sum3/1
  Logical Operator5/1 -> Logical Operator6/2
  [RLceHAD] -> SDelay49/1
  Selector2/1 -> L GLU Golgi Tendon Organs2/1
  Logical Operator4/1 -> Logical Operator7/2
  [LLceHAB] -> SDelay45/1
  Constant4/1 -> R Stance Phase (coronal)/1
  [RonL] -> Logical Operator7/1
  Logical Operator6/1 -> R Swing Phase (coronal)/Enable
  L Swing Phase (coronal)/1 -> "L Stance, Swing, Trans (coronal)"/10, Sum2/1
  L Stance Phase (coronal)/1 -> "L Stance, Swing, Trans (coronal)"/6
  SDelay32/1 -> "L Stance, Swing, Trans (coronal)"/4
  L GLU Golgi Tendon Organs1/1 -> LL Delay6/1
  Sum3/1 -> SDelay43/1
  "L Stance, Swing, Trans (coronal)"/1 -> Saturation3/1
  SDelay43/1 -> L Swing Phase (coronal)/1
  SDelay40/1 -> [LStimHAD]
  MDelay24/1 -> "L Stance, Swing, Trans (coronal)"/1
  Selector1/1 -> Sum5/1
  L Stance afferent delay1/1 -> L Stance Phase (coronal)/Enable, Logical Operator4/1
  SDelay46/1 -> [LStimHAB]
  SDelay45/1 -> L Swing Phase (coronal)/3
  SDelay44/1 -> L Swing Phase (coronal)/2
  [RStance] -> MDelay23/1
  MDelay23/1 -> "R Stance, Swing, Trans (coronal)"/1
  SDelay49/1 -> R Swing Phase (coronal)/2
  [R_LHSwStim] -> R Stance Phase (coronal)/3
  Logical Operator7/1 -> L Swing Phase (coronal)/Enable
  Sum2/1 -> [R_LHSwStim]
  [LStance] -> L Stance afferent delay1/1
  L Stance Phase (coronal)/4 -> "L Stance, Swing, Trans (coronal)"/9
  Demux1/2 -> SDelay37/1
  SDelay42/1 -> L Stance Phase (coronal)/2
  [RonL] -> "L Stance, Swing, Trans (coronal)"/3
  L Stance afferent delay2/1 -> R Stance Phase (coronal)/Enable, Logical Operator5/1
  L Stance Phase (coronal)/3 -> "L Stance, Swing, Trans (coronal)"/8
  SDelay36/1 -> "L Stance, Swing, Trans (coronal)"/5
  Demux2/1 -> SDelay46/1
  [LLLoad] -> SDelay32/1
  [RStance] -> MDelay21/1
  [RLLoad] -> SDelay33/1
  [RStance] -> L Stance afferent delay2/1
  [LStance] -> MDelay24/1
  [LLLoad] -> SDelay41/1
  [LonR] -> Logical Operator6/1
  [RLLoad] -> SDelay36/1
  [R_RHSwStim] -> L Stance Phase (coronal)/3
  L GLU Golgi Tendon Organs3/1 -> L Stance Phase (coronal)/1
  SDelay41/1 -> "R Stance, Swing, Trans (coronal)"/5
  "R Stance, Swing, Trans (coronal)"/1 -> Saturation2/1
  SDelay47/1 -> R Stance Phase (coronal)/2
  Constant2/1 -> Sum5/3
  R Stance Phase (coronal)/2 -> "R Stance, Swing, Trans (coronal)"/7
  SDelay38/1 -> R Stance Phase (coronal)/4
  Saturation2/1 -> Demux1/1
  [LStance] -> MDelay22/1
  SDelay34/1 -> R Swing Phase (coronal)/3
  MDelay22/1 -> "R Stance, Swing, Trans (coronal)"/2
  Constant1/1 -> Sum3/3
  [LonR] -> "R Stance, Swing, Trans (coronal)"/3
  SDelay48/1 -> R Swing Phase (coronal)/1
  [RLceHAB] -> SDelay34/1
  R Stance Phase (coronal)/1 -> "R Stance, Swing, Trans (coronal)"/6
  Saturation3/1 -> Demux2/1
  R Swing Phase (coronal)/1 -> "R Stance, Swing, Trans (coronal)"/10, Sum4/1
  LL Delay7/1 -> SDelay47/1
  R Stance Phase (coronal)/3 -> "R Stance, Swing, Trans (coronal)"/8
  LL Delay6/1 -> SDelay42/1
  R Stance Phase (coronal)/4 -> "R Stance, Swing, Trans (coronal)"/9
  Demux1/1 -> SDelay35/1
  Demux2/2 -> SDelay40/1
  R Swing Phase (coronal)/2 -> "R Stance, Swing, Trans (coronal)"/11, Sum4/2
  SDelay33/1 -> "R Stance, Swing, Trans (coronal)"/4
  Sum4/1 -> [R_RHSwStim]
  [RhipR_tgt] -> Sum5/2
  Constant3/1 -> L GLU Golgi Tendon Organs3/1
  "L Stance, Swing, Trans (sagittal)"/1 -> Saturation10/1
  [RphiANDdphiHip] -> Right Hard Stops/2
  Demux10/2 -> [RKneeMoment]
  [RphiANDdphiAnkle] -> Right Hard Stops/4
  [LMuscleTorques] -> Scope3/1, Left Hard Stops/1
  [LphiANDdphiAnkle] -> Left Hard Stops/4
  [LphiANDdphiKnee] -> Left Hard Stops/3
  [RMuscleTorques] -> Scope4/1, Right Hard Stops/1
  [LphiANDdphiHip] -> Left Hard Stops/2
  Right Hard Stops/1 -> Demux10/1
  Left Hard Stops/1 -> Demux8/1
  Right Hard Stops/3 -> Scope2/2, [RKneeStopMoment]
  Demux10/1 -> [RHipMoment]
  Demux10/3 -> [RAnkleMoment]
  Left Hard Stops/4 -> Scope1/3, [LAnkleStopMoment]
  Right Hard Stops/2 -> Scope2/1, [RHipStopMoment]
  Left Hard Stops/3 -> [LKneeStopMoment], Scope1/2
  Right Hard Stops/4 -> [RAnkleStopMoment], Scope2/3
  Demux8/2 -> [LKneeMoment]
  Left Hard Stops/2 -> Scope1/1, [LHipStopMoment]
  Demux8/1 -> [LHipMoment]
  Demux8/3 -> [LAnkleMoment]
  [RphiANDdphiKnee] -> Right Hard Stops/3
  [LMuscleTorquesR] -> Left Hard Stops/5
  [RMuscleTorquesR] -> Right Hard Stops/5
  Left Hard Stops/5 -> [LHipMomentR]
  Right Hard Stops/5 -> [RHipMomentR]
  [LthetaANDdthetaHipR] -> Left Hard Stops/6
  [RthetaANDdthetaHipR] -> Right Hard Stops/6
  Left Hard Stops/6 -> [LHipRStopMoment]
  Right Hard Stops/6 -> [RHipRStopMoment]
  [phiANDdphiHAT] -> Selector/1
  [thetaANDdthetaHAT] -> LL Delay7/1, Selector1/1
  [thetaANDdthetaHAT] -> L GLU Golgi Tendon Organs1/1, Selector2/1
  [LStance] -> L Swing Phase (sagittal)/1, L Stance afferent delay/1
  [RStance] -> R Stance afferent delay/1
  Sum5/1 -> SDelay48/1
